simulink model "DisplayCustomization"  (R2020b)
settings: Solver=VariableStepAuto  StartTime=0.0  StopTime=10.0  RelTol=1e-3
settings Model: Creator=macra  LastModifiedBy=macra

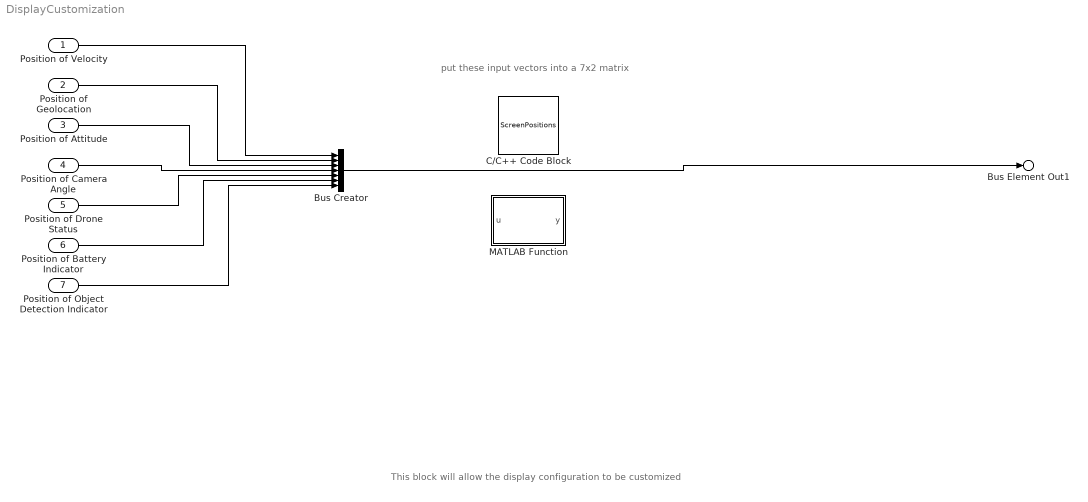
== system DisplayCustomization ==
  note: put these input vectors into a 7x2 matrix
  note: This block will allow the display configuration to be customized
  Position of Velocity : Inport  OutDataTypeStr=int16  PortDimensions=[1 1]
  Position of Geolocation : Inport  Port=2  OutDataTypeStr=int16  PortDimensions=[1 1]
  Position of Attitude : Inport  Port=3  OutDataTypeStr=int16  PortDimensions=[1 1]
  Position of Camera Angle : Inport  Port=4  OutDataTypeStr=int16  PortDimensions=[1 1]
  Position of Drone Status : Inport  Port=5  OutDataTypeStr=int16  PortDimensions=[1 1]
  Position of Battery Indicator : Inport  Port=6  OutDataTypeStr=int16  PortDimensions=[1 1]
  Position of Object Detection Indicator : Inport  Port=7  OutDataTypeStr=int16  PortDimensions=[1 1]
  Bus Creator : BusCreator  Inputs=7
  C/C++ Code Block : S-Function  FunctionName=ScreenPositions  SFunctionDeploymentMode=off  EnableBusSupport=off  mask(S-Function Builder){}
      mask help: Simulink:masks:SFunctionBuilder_MD
      mask init:
      | val = [[.9  0.75 0.75 1 1 .9 .9 1]',[1 1 0.75 0.75 .9 .9 1 .9]'];try , sys = get_param(gcb,'SfunBuilderFcnName');if isempty(sys), sys = get_param(gcb,'FunctionName'); end,catch, sys = get_param(gcb,'FunctionName'); end
      settings: CopyFcn=set_param(gcbh,'LinkStatus','none')  OpenFcn=sfunctionwizard(gcbh)
      mask Display: plot(val(:,1),val(:,2)),disp(sys),port_label('input',1,'u0'),port_label('output',1,'y0')
  MATLAB Function : MATLAB Function  TreatAsAtomicUnit=on
  Bus Element Out1 : Outport  PortName=Screen Postions of Data
  wires:
  Bus Creator/1 -> Bus Element Out1/1
  Position of Object Detection Indicator/1 -> Bus Creator/7
  Position of Velocity/1 -> Bus Creator/1
  Position of Geolocation/1 -> Bus Creator/2
  Position of Battery Indicator/1 -> Bus Creator/6
  Position of Drone Status/1 -> Bus Creator/5
  Position of Attitude/1 -> Bus Creator/3
  Position of Camera Angle/1 -> Bus Creator/4

== matlab function DisplayCustomization/MATLAB Function ==
  data: u input; y output
function y = fcn(u)

y = u;
